simulink model "receiver_overall_v3"  (Simulink 7.5)
settings: Solver=FixedStepDiscrete  SolverMode=SingleTasking  StartTime=0.0  StopTime=(length(simin.signals.values)-1)/Fs  FixedStep=1  RelTol=1e-3
undefined symbols (not defined in the file): Fs
libraries: xbsIndex_r4 x939, symbols x8, dspsigops x2
(part 1 of 9)
settings Model: Creator=ich  LastModifiedBy=ich
settings DataIOCC: ExternalInput=simin  LimitDataPoints=off  LoadExternalInput=on

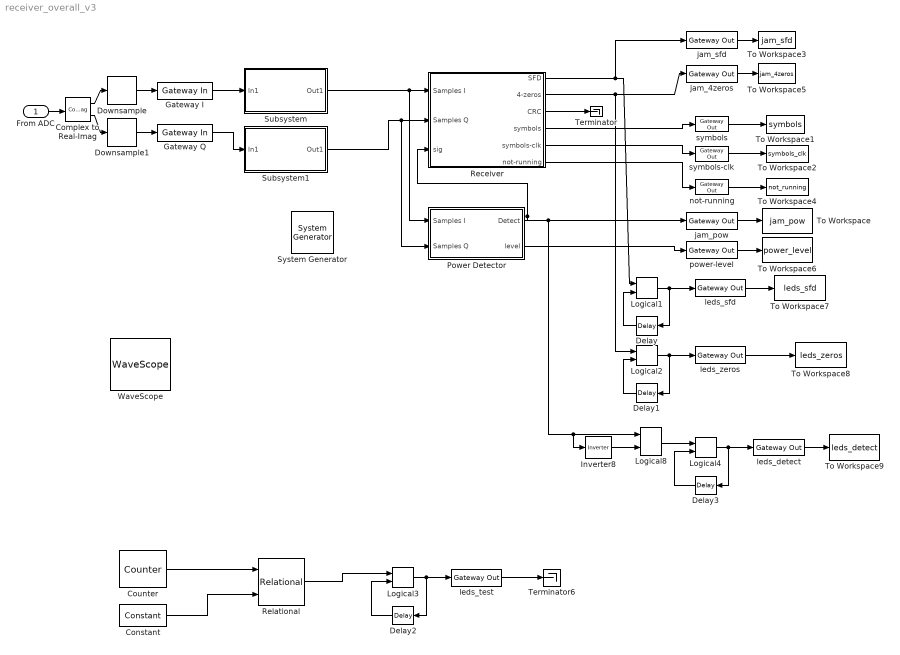
== system receiver_overall_v3 ==
  From ADC : Inport  SampleTime=1/Fs  OutDataType=fixdt(1, 16)  OutScaling=2^0  Interpolate=off
      settings: SignalType=complex
  " System Generator" : xbsIndex_r4/ System Generator  Tag=genX  SystemSampleTime=-1  xilinxfamily=spartan3  part=xc3s2000  speed=-5  package=fg456  synthesis_tool=XST  clock_wrapper=Clock Enables  directory=G:/Projekte/wireless_firewall/dschung/IEEE 802.15.4 receiver/receiver_v3  testbench=off  simulink_period=1  sysclk_period=10  dcm_input_clock_period=10  incr_netlist=off  trim_vbits=Everywhere in SubSystem  dbl_ovrd=According to Block Masks  core_generation=According to Block Masks  run_coregen=off  deprecated_control=off  eval_field=0  block_type=sysgen
      settings: block_version=12.1
  Complex to Real-Imag : ComplexToRealImag
  Constant : xbsIndex_r4/Constant  arith_type=Unsigned  const=0  n_bits=1  bin_pt=0  explicit_period=off  period=1  equ=P=C  opselect=C  inp2=PCIN>>17  opr=+  inp1=P  carry=CIN  dbl_ovrd=off  block_type=constant
      settings: block_version=12.2
  Counter : xbsIndex_r4/Counter  cnt_type=Count Limited  cnt_to=200000000  operation=Up  start_count=0  cnt_by_val=1  arith_type=Unsigned  n_bits=32  bin_pt=0  load_pin=off  rst=off  en=off  explicit_period=on  period=1  dbl_ovrd=off  use_behavioral_HDL=off  implementation=Fabric  block_type=counter
      settings: block_version=12.2
  Delay{,1..3} (4 alike) : xbsIndex_r4/Delay  en=off  latency=1  dbl_ovrd=off  reg_retiming=off  block_type=delay
      settings: block_version=12.2
  Downsample : dspsigops/Downsample  N=4  phase=0  ic=0  smode=Force single rate  fmode=Maintain input frame size
  Downsample1 : dspsigops/Downsample  N=4  phase=0  ic=0  smode=Force single rate  fmode=Maintain input frame size
  Gateway I : xbsIndex_r4/Gateway In  arith_type="Signed  (2's comp)"  n_bits=15  bin_pt=13  quantization="Round  (unbiased: +/- Inf)"  overflow=Saturate  period=1/Fs  dbl_ovrd=off  timing_constraint=None  locs_specified=off  LOCs={}  hdl_port=on  block_type=gatewayin
      settings: infoedit="Gateway in block.  Converts inputs of type Simulink integer, double and fixed point to  Xilinx fixed point type.<br><br>Hardware notes:  In hardware these blocks become top level input ports."  xl_area=[0 0 0 0 16 0 0]  block_version=12.1
  Gateway Q : xbsIndex_r4/Gateway In  arith_type="Signed  (2's comp)"  n_bits=15  bin_pt=13  quantization="Round  (unbiased: +/- Inf)"  overflow=Saturate  period=1/Fs  dbl_ovrd=off  timing_constraint=None  locs_specified=off  LOCs={}  hdl_port=on  block_type=gatewayin
      settings: infoedit="Gateway in block.  Converts inputs of type Simulink integer, double and fixed point to  Xilinx fixed point type.<br><br>Hardware notes:  In hardware these blocks become top level input ports."  xl_area=[0 0 0 0 16 0 0]  block_version=12.1
  Inverter8 : xbsIndex_r4/Inverter  en=off  latency=1  dbl_ovrd=off  block_type=inv
      settings: block_version=12.2
  Logical{1..4} (4 alike) : xbsIndex_r4/Logical  logical_function=XOR  inputs=2  en=off  latency=0  precision=Full  arith_type=Unsigned  n_bits=16  bin_pt=0  align_bp=on  dbl_ovrd=off  block_type=logical
      settings: block_version=12.2
  Logical8 : xbsIndex_r4/Logical  logical_function=AND  inputs=2  en=off  latency=0  precision=Full  arith_type=Unsigned  n_bits=16  bin_pt=0  align_bp=on  dbl_ovrd=off  block_type=logical
      settings: block_version=12.2
  Power Detector : Subsystem
  Receiver : Subsystem
  Relational : xbsIndex_r4/Relational  mode=a=b  en=off  latency=1  dbl_ovrd=off  block_type=relational
      settings: block_version=12.2
  Subsystem : Subsystem
      mask Display:
      | disp('Interpolate');
      | port_label('input',1,'in');
      | port_label('output',1,'out');
  Subsystem1 : Subsystem
      mask Display:
      | disp('Interpolate');
      | port_label('input',1,'in');
      | port_label('output',1,'out');
  Terminator : Terminator
  Terminator6 : Terminator
  To Workspace : ToWorkspace  VariableName=jam_pow  SampleTime=-1  SaveFormat=Structure
  To Workspace1 : ToWorkspace  VariableName=symbols  SampleTime=-1  SaveFormat=Structure
  To Workspace2 : ToWorkspace  VariableName=symbols_clk  SampleTime=-1  SaveFormat=Structure
  To Workspace3 : ToWorkspace  VariableName=jam_sfd  SampleTime=-1  SaveFormat=Structure
  To Workspace4 : ToWorkspace  VariableName=not_running  SampleTime=-1  SaveFormat=Structure
  To Workspace5 : ToWorkspace  VariableName=jam_4zeros  SampleTime=-1  SaveFormat=Structure
  To Workspace6 : ToWorkspace  VariableName=power_level  SampleTime=-1  SaveFormat=Structure
  To Workspace7 : ToWorkspace  VariableName=leds_sfd  SampleTime=-1  SaveFormat=Structure
  To Workspace8 : ToWorkspace  VariableName=leds_zeros  SampleTime=-1  SaveFormat=Structure
  To Workspace9 : ToWorkspace  VariableName=leds_detect  SampleTime=-1  SaveFormat=Structure
  WaveScope : xbsIndex_r4/WaveScope  block_type=wavescope
      settings: block_version=12.2
  jam_4zeros : xbsIndex_r4/Gateway Out  hdl_port=on  timing_constraint=None  locs_specified=off  LOCs={}  block_type=gatewayout
      settings: infoedit="Gateway out block.  Converts Xilinx fixed point inputs into ouputs of type Simulink integer, double, or fixed point.<br><br>Hardware notes:  In hardware these blocks become top level output ports or are discarded, depending on how they are configured."  block_version=12.2
  jam_pow : xbsIndex_r4/Gateway Out  hdl_port=on  timing_constraint=None  locs_specified=off  LOCs={}  block_type=gatewayout
      settings: infoedit="Gateway out block.  Converts Xilinx fixed point inputs into ouputs of type Simulink integer, double, or fixed point.<br><br>Hardware notes:  In hardware these blocks become top level output ports or are discarded, depending on how they are configured."  block_version=12.2
  jam_sfd : xbsIndex_r4/Gateway Out  hdl_port=on  timing_constraint=None  locs_specified=off  LOCs={}  block_type=gatewayout
      settings: infoedit="Gateway out block.  Converts Xilinx fixed point inputs into ouputs of type Simulink integer, double, or fixed point.<br><br>Hardware notes:  In hardware these blocks become top level output ports or are discarded, depending on how they are configured."  block_version=12.2
  leds_detect : xbsIndex_r4/Gateway Out  hdl_port=on  timing_constraint=None  locs_specified=off  LOCs={}  block_type=gatewayout
      settings: infoedit="Gateway out block.  Converts Xilinx fixed point inputs into ouputs of type Simulink integer, double, or fixed point.<br><br>Hardware notes:  In hardware these blocks become top level output ports or are discarded, depending on how they are configured."  block_version=12.2
  leds_sfd : xbsIndex_r4/Gateway Out  hdl_port=on  timing_constraint=None  locs_specified=off  LOCs={}  block_type=gatewayout
      settings: infoedit="Gateway out block.  Converts Xilinx fixed point inputs into ouputs of type Simulink integer, double, or fixed point.<br><br>Hardware notes:  In hardware these blocks become top level output ports or are discarded, depending on how they are configured."  block_version=12.2
  leds_test : xbsIndex_r4/Gateway Out  hdl_port=on  timing_constraint=None  locs_specified=off  LOCs={}  block_type=gatewayout
      settings: infoedit="Gateway out block.  Converts Xilinx fixed point inputs into ouputs of type Simulink integer, double, or fixed point.<br><br>Hardware notes:  In hardware these blocks become top level output ports or are discarded, depending on how they are configured."  block_version=12.2
  leds_zeros : xbsIndex_r4/Gateway Out  hdl_port=on  timing_constraint=None  locs_specified=off  LOCs={}  block_type=gatewayout
      settings: infoedit="Gateway out block.  Converts Xilinx fixed point inputs into ouputs of type Simulink integer, double, or fixed point.<br><br>Hardware notes:  In hardware these blocks become top level output ports or are discarded, depending on how they are configured."  block_version=12.2
  not-running : xbsIndex_r4/Gateway Out  hdl_port=on  timing_constraint=None  locs_specified=off  LOCs={}  block_type=gatewayout
      settings: infoedit="Gateway out block.  Converts Xilinx fixed point inputs into ouputs of type Simulink integer, double, or fixed point.<br><br>Hardware notes:  In hardware these blocks become top level output ports or are discarded, depending on how they are configured."  block_version=12.2
  power-level : xbsIndex_r4/Gateway Out  hdl_port=on  timing_constraint=None  locs_specified=off  LOCs={}  block_type=gatewayout
      settings: infoedit="Gateway out block.  Converts Xilinx fixed point inputs into ouputs of type Simulink integer, double, or fixed point.<br><br>Hardware notes:  In hardware these blocks become top level output ports or are discarded, depending on how they are configured."  block_version=12.2
  symbols : xbsIndex_r4/Gateway Out  hdl_port=on  timing_constraint=None  locs_specified=off  LOCs={}  block_type=gatewayout
      settings: infoedit="Gateway out block.  Converts Xilinx fixed point inputs into ouputs of type Simulink integer, double, or fixed point.<br><br>Hardware notes:  In hardware these blocks become top level output ports or are discarded, depending on how they are configured."  block_version=12.2
  symbols-clk : xbsIndex_r4/Gateway Out  hdl_port=on  timing_constraint=None  locs_specified=off  LOCs={}  block_type=gatewayout
      settings: infoedit="Gateway out block.  Converts Xilinx fixed point inputs into ouputs of type Simulink integer, double, or fixed point.<br><br>Hardware notes:  In hardware these blocks become top level output ports or are discarded, depending on how they are configured."  block_version=12.2
  wires:
  Gateway I/1 -> Subsystem/1(In1)
  Gateway Q/1 -> Subsystem1/1(In1)
  From ADC/1 -> Complex to Real-Imag/1
  Complex to Real-Imag/1 -> Downsample/1
  Complex to Real-Imag/2 -> Downsample1/1
  Receiver/3(CRC) -> Terminator/1
  Logical1/1 -> Delay/1, leds_sfd/1
  Delay/1 -> Logical1/2
  Logical2/1 -> Delay1/1, leds_zeros/1
  Delay1/1 -> Logical2/2
  leds_test/1 -> Terminator6/1
  Logical3/1 -> Delay2/1, leds_test/1
  Delay2/1 -> Logical3/2
  Counter/1 -> Relational/1
  Constant/1 -> Relational/2
  Relational/1 -> Logical3/1
  symbols/1 -> To Workspace1/1
  symbols-clk/1 -> To Workspace2/1
  Receiver/2(4-zeros) -> Logical2/1, jam_4zeros/1
  Receiver/1(SFD) -> Logical1/1, jam_sfd/1
  Receiver/4(symbols) -> symbols/1
  Receiver/5(symbols-clk) -> symbols-clk/1
  not-running/1 -> To Workspace4/1
  Receiver/6(not-running) -> not-running/1
  jam_4zeros/1 -> To Workspace5/1
  jam_sfd/1 -> To Workspace3/1
  Power Detector/1(Detect) -> Receiver/3(sig), jam_pow/1, Logical8/1, Inverter8/1
  jam_pow/1 -> To Workspace/1
  power-level/1 -> To Workspace6/1
  Power Detector/2(level) -> power-level/1
  Subsystem/1(Out1) -> Receiver/1(Samples I), Power Detector/1(Samples I)
  Subsystem1/1(Out1) -> Receiver/2(Samples Q), Power Detector/2(Samples Q)
  Downsample/1 -> Gateway I/1
  Downsample1/1 -> Gateway Q/1
  leds_sfd/1 -> To Workspace7/1
  leds_zeros/1 -> To Workspace8/1
  Inverter8/1 -> Logical8/2
  Logical4/1 -> Delay3/1, leds_detect/1
  Logical8/1 -> Logical4/1
  Delay3/1 -> Logical4/2
  leds_detect/1 -> To Workspace9/1

== system receiver_overall_v3/Power Detector ==
  note: 14bit signed * 14bit signed = 29bit unsigned
      | but one bit only for 10...0 * 10...0 is too expensive -> 28bit
  Samples I : Inport
  Samples Q : Inport  Port=2
  -3dB : xbsIndex_r4/Constant  arith_type=Unsigned  const=0.5  n_bits=16  bin_pt=16  explicit_period=off  period=1  equ=P=C  opselect=C  inp2=PCIN>>17  opr=+  inp1=P  carry=CIN  dbl_ovrd=off  block_type=constant
      settings: block_version=12.2
  AddSub : xbsIndex_r4/AddSub  mode=Addition  use_carryin=off  use_carryout=off  en=off  latency=0  precision=Full  arith_type=Unsigned  n_bits=16  bin_pt=14  quantization=Truncate  overflow=Wrap  dbl_ovrd=off  use_behavioral_HDL=off  hw_selection=Fabric  pipelined=off  block_type=addsub
      settings: block_version=12.2
  Convert : xbsIndex_r4/Convert  arith_type="Signed  (2's comp)"  n_bits=14  bin_pt=12  quantization=Truncate  overflow=Wrap  en=off  latency=0  dbl_ovrd=off  pipeline=off  block_type=convert
      settings: block_version=12.2
  Convert1 : xbsIndex_r4/Convert  arith_type="Signed  (2's comp)"  n_bits=14  bin_pt=12  quantization=Truncate  overflow=Wrap  en=off  latency=0  dbl_ovrd=off  pipeline=off  block_type=convert
      settings: block_version=12.2
  Moving Average : Subsystem
  Mult : xbsIndex_r4/Mult  precision=User Defined  arith_type=Unsigned  n_bits=28  bin_pt=26  quantization=Truncate  overflow=Wrap  en=off  latency=4  dbl_ovrd=off  use_behavioral_HDL=off  opt=Speed  use_embedded=off  optimum_pipeline=on  pipeline=on  use_rpm=on  placement_style=Triangular  block_type=mult
      settings: block_version=12.2
  Mult1 : xbsIndex_r4/Mult  precision=User Defined  arith_type=Unsigned  n_bits=28  bin_pt=26  quantization=Truncate  overflow=Wrap  en=off  latency=4  dbl_ovrd=off  use_behavioral_HDL=off  opt=Speed  use_embedded=off  optimum_pipeline=on  pipeline=on  use_rpm=on  placement_style=Triangular  block_type=mult
      settings: block_version=12.2
  Relational2 : xbsIndex_r4/Relational  mode=a>b  en=off  latency=1  dbl_ovrd=off  block_type=relational
      settings: block_version=12.2
  Detect : Outport
  level : Outport  Port=2
  wires:
  Samples Q/1 -> Convert1/1
  Relational2/1 -> Detect/1
  Samples I/1 -> Convert/1
  Mult/1 -> AddSub/1
  Mult1/1 -> AddSub/2
  AddSub/1 -> Moving Average/1(in)
  -3dB/1 -> Relational2/2
  Moving Average/1(short) -> Relational2/1, level/1
  Convert/1 -> Mult/1, Mult/2
  Convert1/1 -> Mult1/2, Mult1/1

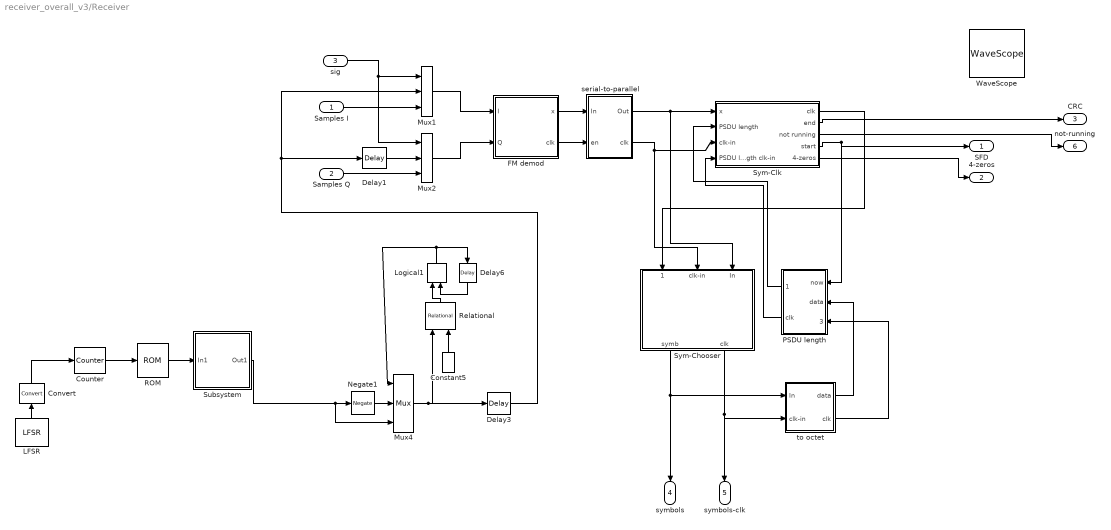
== system receiver_overall_v3/Receiver ==
  Samples I : Inport  SampleTime=1/Fs  OutDataType=fixdt(1, 16)  OutScaling=2^0  Interpolate=off
  Samples Q : Inport  Port=2  SampleTime=1/Fs  OutDataType=fixdt(1, 16)  OutScaling=2^0  Interpolate=off
  sig : Inport  Port=3  OutDataType=fixdt(1, 16)  OutScaling=2^0
  Constant5 : xbsIndex_r4/Constant  arith_type=Unsigned  const=0  n_bits=1  bin_pt=0  explicit_period=on  period=1  equ=P=C  opselect=C  inp2=PCIN>>17  opr=+  inp1=P  carry=CIN  dbl_ovrd=off  block_type=constant
      settings: block_version=12.2
  Convert : xbsIndex_r4/Convert  arith_type=Boolean  n_bits=16  bin_pt=14  quantization=Truncate  overflow=Wrap  en=off  latency=0  dbl_ovrd=off  pipeline=off  block_type=convert
      settings: block_version=12.2
  Counter : xbsIndex_r4/Counter  cnt_type=Count Limited  cnt_to=24  operation=Up  start_count=0  cnt_by_val=1  arith_type=Unsigned  n_bits=5  bin_pt=0  load_pin=off  rst=off  en=on  explicit_period=on  period=1  dbl_ovrd=off  use_behavioral_HDL=off  implementation=Fabric  block_type=counter
      settings: block_version=12.2
  Delay1 : xbsIndex_r4/Delay  en=off  latency=50  dbl_ovrd=off  reg_retiming=off  block_type=delay
      settings: block_version=12.2
  Delay3 : xbsIndex_r4/Delay  en=off  latency=30  dbl_ovrd=off  reg_retiming=off  block_type=delay
      settings: block_version=12.2
  Delay6 : xbsIndex_r4/Delay  en=off  latency=1  dbl_ovrd=off  reg_retiming=off  block_type=delay
      settings: block_version=12.2
  FM demod : Subsystem
      mask Display:
      | disp('FM\ndemod');
      | port_label('input',1,'I');
      | port_label('input',2,'Q');
      | port_label('output',1,'x');
      | port_label('output',2,'clk');
  LFSR : xbsIndex_r4/LFSR  lfsr_type=Fibonacci  gate_type=XOR  n_bits=4  polynomial='1'  rst_value='1'  rst=off  en=off  reloadable_seed=off  input_type=off  output_type=off  arith_type="Signed  (2's comp)"  bin_pt=4  dbl_ovrd=off  explicit_period=off  period=1  block_type=lfsr
      settings: block_version=12.2
  Logical1 : xbsIndex_r4/Logical  logical_function=XOR  inputs=2  en=off  latency=0  precision=Full  arith_type=Unsigned  n_bits=16  bin_pt=0  align_bp=on  dbl_ovrd=off  block_type=logical
      settings: block_version=12.2
  Mux1 : xbsIndex_r4/Mux  inputs=2  en=off  latency=0  precision=User Defined  arith_type="Signed  (2's comp)"  n_bits=15  bin_pt=13  quantization=Truncate  overflow=Wrap  dbl_ovrd=off  block_type=mux
      settings: block_version=12.2
  Mux2 : xbsIndex_r4/Mux  inputs=2  en=off  latency=0  precision=User Defined  arith_type="Signed  (2's comp)"  n_bits=15  bin_pt=13  quantization=Truncate  overflow=Wrap  dbl_ovrd=off  block_type=mux
      settings: block_version=12.2
  Mux4 : xbsIndex_r4/Mux  inputs=2  en=off  latency=0  precision=Full  arith_type=Unsigned  n_bits=16  bin_pt=14  quantization=Truncate  overflow=Wrap  dbl_ovrd=off  block_type=mux
      settings: block_version=12.2
  Negate1 : xbsIndex_r4/Negate  precision=Full  arith_type="Signed  (2's comp)"  n_bits=16  bin_pt=14  quantization=Truncate  overflow=Wrap  en=off  latency=0  dbl_ovrd=off  block_type=negate
      settings: block_version=12.2
  PSDU length : Subsystem
  ROM : xbsIndex_r4/ROM  depth=25  initVector=sin(pi*(0:4:99)/100)  distributed_mem=Distributed memory  rst=off  init_reg=0  en=off  latency=2  arith_type=Unsigned  n_bits=14  bin_pt=13  dbl_ovrd=off  optimize=Area  use_rpm=on  block_type=sprom
      settings: block_version=12.2
  Relational : xbsIndex_r4/Relational  mode=a=b  en=off  latency=1  dbl_ovrd=off  block_type=relational
      settings: block_version=12.2
  Subsystem : Subsystem
      mask Display:
      | disp('Interpolate');
      | port_label('input',1,'in');
      | port_label('output',1,'out');
  Sym-Chooser : Subsystem
  Sym-Clk : Subsystem
  WaveScope : xbsIndex_r4/WaveScope  block_type=wavescope
      settings: block_version=12.2
  serial-to-parallel : Subsystem
      mask init:
      | % save_gcb = gcb
      | % nbits=bits+1
      | % old=find_system(save_gcb,...
      | %     'lookUnderMasks', 'all',...
      | %     'RegExp', 'On',...
      | %     'Name', 'DE\d+');
      | % 
      | %     for i=1:length(old)-1
      | %         delete_line(gcb, ['DE' int2str(i) '/1'], ['DE' int2str(i+1) '/1']);
      | %     end
      | %     for i=1:length(old)
      | %         delete_line(gcb, ['DE' int2str(i) '/2'], ['Concat/' int2str(length(old)-i+1)]);
      | %     end
      | %     delete_line(gcb, '1to2/2', ['Concat/', int2str(length(old)+1)]);
      | %     delete_line(gcb, ['DE' int2str(length(old)) '/1'], ['Terminator/1']);
      | %     for i=2:length(old)
      | %         delete_block(old{i});
      | %     end
      | % 
      | % pos = get_param([save_gcb '/DE1'], 'Position');
      | % width = pos(3)-pos(1);
      | % for i=3:nbits,
      | %     add_block([save_gcb '/DE1'],[save_gcb '/DE' int2str(i-1)],'position',[pos(1)+2*(i-2)*width, pos(2), pos(3)+2*(i-2)*width, pos(4)]);
      | %     add_line(save_gcb, ['DE' int2str(i-2) '/1'], ['DE' int2str(i-1) '/1'], 'autorouting', 'on');    
      | % end
      | % 
      | % posT = get_param([save_gcb '/Terminator'], 'Position');
      | % widthT = posT(3)-posT(1);
      | % heightT = posT(4)-posT(2);
      | % set_param([save_gcb '/Terminator'], 'Position', [pos(1)+2*(nbits-1)*width pos(2) pos(1)+2*(nbits-1)*width+widthT pos(2)+heightT]);
      | % 
      | % add_line(save_gcb, ['DE' int2str(nbits-1) '/1'], ['Terminator/1'], 'autorouting', 'on');
      | % 
      | % posC = get_param([save_gcb '/Concat'], 'Position');
      | % set_param([save_gcb '/Concat'], 'Position', [pos(1)+2*(nbits)*width posC(2) pos(1)+2*(nbits+1)*width posC(2)+2*(nbits-1)*width]);
      | % set_param([save_gcb '/Concat'], 'num_inputs', int2str(nbits));
      | % 
      | % add_line(save_gcb, '1to2/2', ['Concat/' int2str(nbits)], 'autorouting', 'on');
      | % for i=1:nbits-1,
      | %    add_line(save_gcb, ['DE' int2str(i) '/2'], ['Concat/' int2str(nbits-i)], 'autorouting', 'on');
      | % end
  to octet : Subsystem
  SFD : Outport  OutDataType=fixdt(1, 16)  OutScaling=2^0
  4-zeros : Outport  Port=2  OutDataType=fixdt(1, 16)  OutScaling=2^0
  CRC : Outport  Port=3  OutDataType=fixdt(1, 16)  OutScaling=2^0
  symbols : Outport  Port=4  OutDataType=fixdt(1, 16)  OutScaling=2^0
  symbols-clk : Outport  Port=5  OutDataType=fixdt(1, 16)  OutScaling=2^0
  not-running : Outport  Port=6  OutDataType=fixdt(1, 16)  OutScaling=2^0
  wires:
  Sym-Clk/1(clk) -> Sym-Chooser/1(clk-symb-in)
  PSDU length/1(length) -> Sym-Clk/2(PSDU length)
  Sym-Clk/2(end) -> CRC/1
  Sym-Chooser/1(symb) -> to octet/1(In), symbols/1
  FM demod/1(x) -> serial-to-parallel/1(In)
  serial-to-parallel/1(Out) -> Sym-Clk/1(x), Sym-Chooser/3(In)
  Sym-Clk/4(start) -> PSDU length/1(now), SFD/1
  Sym-Clk/3(not running) -> not-running/1
  FM demod/2(clk) -> serial-to-parallel/2(en)
  serial-to-parallel/2(clk) -> Sym-Clk/3(clk-in), Sym-Chooser/2(clk-in)
  Samples I/1 -> Mux1/3
  Samples Q/1 -> Mux2/3
  sig/1 -> Mux1/1, Mux2/1
  Mux1/1 -> FM demod/1(I)
  Mux2/1 -> FM demod/2(Q)
  Sym-Chooser/2(clk) -> to octet/2(clk-in), symbols-clk/1
  to octet/1(data) -> PSDU length/2(data)
  to octet/2(clk) -> PSDU length/3(clk-in)
  PSDU length/2(clk) -> Sym-Clk/4(PSDU length clk-in)
  Sym-Clk/5(4-zeros) -> 4-zeros/1
  Delay1/1 -> Mux2/2
  Counter/1 -> ROM/1
  Subsystem/1(Out1) -> Negate1/1, Mux4/3
  Mux4/1 -> Relational/1, Delay3/1
  Constant5/1 -> Relational/2
  Relational/1 -> Logical1/1
  Logical1/1 -> Delay6/1, Mux4/1
  Delay6/1 -> Logical1/2
  Negate1/1 -> Mux4/2
  LFSR/1 -> Convert/1
  Convert/1 -> Counter/1
  Delay3/1 -> Delay1/1, Mux1/2
  ROM/1 -> Subsystem/1(In1)

== system receiver_overall_v3/Subsystem ==
  In1 : Inport
  AddSub1 : xbsIndex_r4/AddSub  mode=Addition  use_carryin=off  use_carryout=off  en=off  latency=0  precision=Full  arith_type=Unsigned  n_bits=16  bin_pt=14  quantization=Truncate  overflow=Wrap  dbl_ovrd=off  use_behavioral_HDL=off  hw_selection=Fabric  pipelined=off  block_type=addsub
      settings: block_version=12.2
  AddSub2 : xbsIndex_r4/AddSub  mode=Addition  use_carryin=off  use_carryout=off  en=off  latency=0  precision=Full  arith_type=Unsigned  n_bits=16  bin_pt=14  quantization=Truncate  overflow=Wrap  dbl_ovrd=off  use_behavioral_HDL=off  hw_selection=Fabric  pipelined=off  block_type=addsub
      settings: block_version=12.2
  AddSub3 : xbsIndex_r4/AddSub  mode=Addition  use_carryin=off  use_carryout=off  en=off  latency=1  precision=Full  arith_type=Unsigned  n_bits=16  bin_pt=14  quantization=Truncate  overflow=Wrap  dbl_ovrd=off  use_behavioral_HDL=off  hw_selection=Fabric  pipelined=off  block_type=addsub
      settings: block_version=12.2
  Convert : xbsIndex_r4/Convert  arith_type="Signed  (2's comp)"  n_bits=15  bin_pt=13  quantization=Truncate  overflow=Wrap  en=off  latency=0  dbl_ovrd=off  pipeline=off  block_type=convert
      settings: block_version=12.2
  Delay2 : xbsIndex_r4/Delay  en=off  latency=1  dbl_ovrd=off  reg_retiming=off  block_type=delay
      settings: block_version=12.2
  Delay4 : xbsIndex_r4/Delay  en=off  latency=1  dbl_ovrd=off  reg_retiming=off  block_type=delay
      settings: block_version=12.2
  Delay5 : xbsIndex_r4/Delay  en=off  latency=1  dbl_ovrd=off  reg_retiming=off  block_type=delay
      settings: block_version=12.2
  Reinterpret : xbsIndex_r4/Reinterpret  force_arith_type=off  arith_type=Unsigned  force_bin_pt=on  bin_pt=15  block_type=reinterpret
      settings: infoedit="Changes signal type without altering the binary representation.   You can changed the signal between signed and unsigned, and relocate the binary point.<br><br>Hardware notes: In hardware this block costs nothing.<br><br>Example:  Suppose the input is 6 bits wide, signed, with 2 fractional bits, and the output is forced to unsigned with 0 fractional bits.  Then an input of -2.0 (1110.00 in binary 2's complement) becomes an output of 56 (111000 in binary)."  block_version=12.2
  Out1 : Outport
  wires:
  In1/1 -> Delay2/1, AddSub1/1
  Delay2/1 -> AddSub1/2, Delay4/1
  Delay4/1 -> AddSub2/1, Delay5/1
  Delay5/1 -> AddSub2/2
  AddSub1/1 -> AddSub3/1
  AddSub2/1 -> AddSub3/2
  AddSub3/1 -> Reinterpret/1
  Reinterpret/1 -> Convert/1
  Convert/1 -> Out1/1

== system receiver_overall_v3/Subsystem1 ==
  In1 : Inport
  AddSub1 : xbsIndex_r4/AddSub  mode=Addition  use_carryin=off  use_carryout=off  en=off  latency=0  precision=Full  arith_type=Unsigned  n_bits=16  bin_pt=14  quantization=Truncate  overflow=Wrap  dbl_ovrd=off  use_behavioral_HDL=off  hw_selection=Fabric  pipelined=off  block_type=addsub
      settings: block_version=12.2
  AddSub2 : xbsIndex_r4/AddSub  mode=Addition  use_carryin=off  use_carryout=off  en=off  latency=0  precision=Full  arith_type=Unsigned  n_bits=16  bin_pt=14  quantization=Truncate  overflow=Wrap  dbl_ovrd=off  use_behavioral_HDL=off  hw_selection=Fabric  pipelined=off  block_type=addsub
      settings: block_version=12.2
  AddSub3 : xbsIndex_r4/AddSub  mode=Addition  use_carryin=off  use_carryout=off  en=off  latency=1  precision=Full  arith_type=Unsigned  n_bits=16  bin_pt=14  quantization=Truncate  overflow=Wrap  dbl_ovrd=off  use_behavioral_HDL=off  hw_selection=Fabric  pipelined=off  block_type=addsub
      settings: block_version=12.2
  Convert : xbsIndex_r4/Convert  arith_type="Signed  (2's comp)"  n_bits=15  bin_pt=13  quantization=Truncate  overflow=Wrap  en=off  latency=0  dbl_ovrd=off  pipeline=off  block_type=convert
      settings: block_version=12.2
  Delay2 : xbsIndex_r4/Delay  en=off  latency=1  dbl_ovrd=off  reg_retiming=off  block_type=delay
      settings: block_version=12.2
  Delay4 : xbsIndex_r4/Delay  en=off  latency=1  dbl_ovrd=off  reg_retiming=off  block_type=delay
      settings: block_version=12.2
  Delay5 : xbsIndex_r4/Delay  en=off  latency=1  dbl_ovrd=off  reg_retiming=off  block_type=delay
      settings: block_version=12.2
  Reinterpret : xbsIndex_r4/Reinterpret  force_arith_type=off  arith_type=Unsigned  force_bin_pt=on  bin_pt=15  block_type=reinterpret
      settings: infoedit="Changes signal type without altering the binary representation.   You can changed the signal between signed and unsigned, and relocate the binary point.<br><br>Hardware notes: In hardware this block costs nothing.<br><br>Example:  Suppose the input is 6 bits wide, signed, with 2 fractional bits, and the output is forced to unsigned with 0 fractional bits.  Then an input of -2.0 (1110.00 in binary 2's complement) becomes an output of 56 (111000 in binary)."  block_version=12.2
  Out1 : Outport
  wires:
  In1/1 -> Delay2/1, AddSub1/1
  Delay2/1 -> AddSub1/2, Delay4/1
  Delay4/1 -> AddSub2/1, Delay5/1
  Delay5/1 -> AddSub2/2
  AddSub1/1 -> AddSub3/1
  AddSub2/1 -> AddSub3/2
  AddSub3/1 -> Reinterpret/1
  Reinterpret/1 -> Convert/1
  Convert/1 -> Out1/1

== system receiver_overall_v3/Power Detector/Moving Average ==
  in : Inport
  AddSub1 : xbsIndex_r4/AddSub  mode=Addition  use_carryin=off  use_carryout=off  en=off  latency=1  precision=User Defined  arith_type="Signed  (2's comp)"  n_bits=39  bin_pt=31  quantization=Truncate  overflow=Wrap  dbl_ovrd=off  use_behavioral_HDL=off  hw_selection=Fabric  pipelined=off  block_type=addsub
      settings: block_version=12.2
  AddSub2 : xbsIndex_r4/AddSub  mode=Subtraction  use_carryin=off  use_carryout=off  en=off  latency=0  precision=Full  arith_type=Unsigned  n_bits=16  bin_pt=14  quantization=Truncate  overflow=Wrap  dbl_ovrd=off  use_behavioral_HDL=off  hw_selection=Fabric  pipelined=off  block_type=addsub
      settings: block_version=12.2
  Convert : xbsIndex_r4/Convert  arith_type="Signed  (2's comp)"  n_bits=31  bin_pt=31  quantization=Truncate  overflow=Wrap  en=off  latency=0  dbl_ovrd=off  pipeline=off  block_type=convert
      settings: block_version=12.2
  Delay1 : xbsIndex_r4/Delay  en=off  latency=32  dbl_ovrd=off  reg_retiming=off  block_type=delay
      settings: block_version=12.2
  Down Sample : xbsIndex_r4/Down Sample  sample_ratio=6  sample_phase="Last Value of Frame  (most efficient)"  en=off  latency=1  dbl_ovrd=off  block_type=dsamp
      settings: block_version=12.2
  Reinterpret : xbsIndex_r4/Reinterpret  force_arith_type=off  arith_type=Unsigned  force_bin_pt=on  bin_pt=31  block_type=reinterpret
      settings: infoedit="Changes signal type without altering the binary representation.   You can changed the signal between signed and unsigned, and relocate the binary point.<br><br>Hardware notes: In hardware this block costs nothing.<br><br>Example:  Suppose the input is 6 bits wide, signed, with 2 fractional bits, and the output is forced to unsigned with 0 fractional bits.  Then an input of -2.0 (1110.00 in binary 2's complement) becomes an output of 56 (111000 in binary)."  block_version=12.2
  Up Sample : xbsIndex_r4/Up Sample  sample_ratio=6  copy_samples=on  en=off  latency=0  dbl_ovrd=off  block_type=usamp
      settings: block_version=12.2
  short : Outport
  wires:
  in/1 -> Down Sample/1
  Delay1/1 -> AddSub2/2
  AddSub2/1 -> Convert/1
  AddSub1/1 -> Up Sample/1, AddSub1/2
  Reinterpret/1 -> AddSub1/1
  Down Sample/1 -> Delay1/1, AddSub2/1
  Up Sample/1 -> short/1
  Convert/1 -> Reinterpret/1

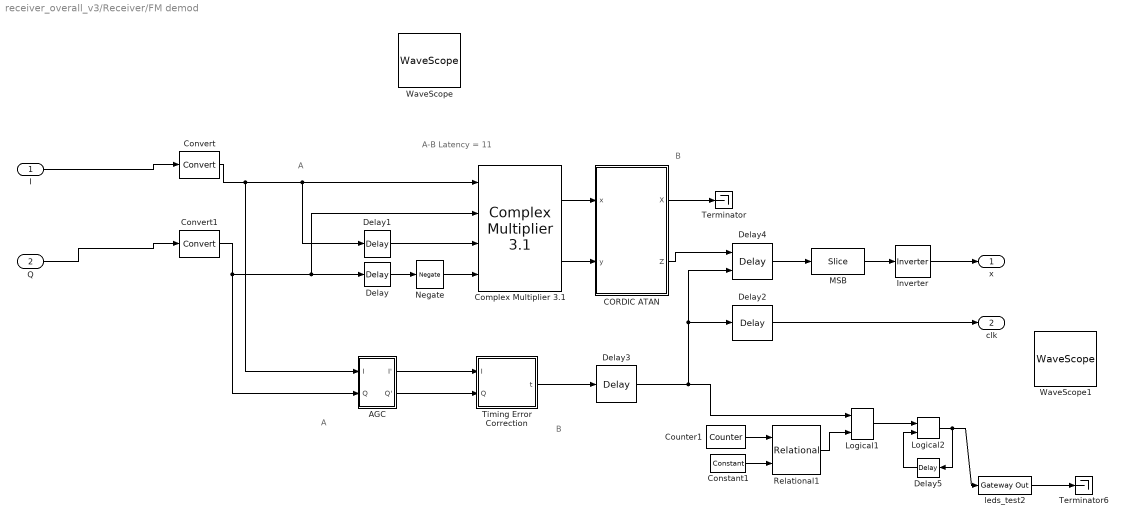
== system receiver_overall_v3/Receiver/FM demod ==
  note: A-B Latency = 11
  note: A
  note: B
  note: A
  note: B
  I : Inport
  Q : Inport  Port=2
  AGC : Subsystem
  CORDIC ATAN : Subsystem  mask(Xilinx CORDIC ATAN){stages=5, pe_nbits=33, pe_binpt=28, pipeline_x=ones(1,5), prev_stages=5, pipeline=[1  1  1  1  1]}
      mask prompts: stages "Number of Processing Elements (integer value starting from 1)"; pe_nbits "X, Y Data Width"; pe_binpt "X, Y Binary Point Position"; pipeline_x "Latency for each Processing Element [1 0 0 1]"; prev_stages "Previous Number of Stages"; pipeline "Previous Pipeline Values"
      mask help: A parallel implementation, circular vectoring mode CORDIC processor for performing rectangular-to-polar conversion. The number of iteration stages (and resultant output accuracy) and the processor arithmetic precision are controlled by the mask customization.
      mask init:
      | [bg,fg] = xlcmap('XBlock',0);
      | iPos = get_param(gcb,'Position');
      | iWidth=iPos(3)-iPos(1); iHeight=iPos(4)-iPos(2);
      | iCx=iWidth/2;
      | iCy=iHeight/2;
      | [logoX, logoY] = xlogo(iPos);
      | sav_gcb=gcb;
      | stages = round(sum(abs(stages)));
      | if (stages == 0)
      | 	stages = prev_stages;
      | end
      | x = zeros(1,stages);
      | pipe_size = max(size(pipeline_x));
      | if pipe_size >= stages
      | 	x(1,1:stages) = pipeline_x(1,1:stages);
      | else
      | 	x(1,1:pipe_size) = pipeline_x(1,1:pipe_size);
      | end
      | 
      | if (stages ~=prev_stages)
      | 	pipeline=x;
      | 	cordic_pe = find_system(gcb, 'lookUnderMasks', 'all', 'FollowLinks','on','masktype', 'CORDIC parallel PE');
      |     
      |   a=find_system(cordic_pe{1}, 'lookUnderMasks', 'all', 'FollowLinks','on','masktype', 'CORDIC iteration PE');
      |   for i= 2:length(a)
      |     for j=1:3
      | 	  delete_line(cordic_pe{1}, ['CORDIC PE' int2str(i-1) '/' int2str(j)], ['CORDIC PE' int2str(i) '/' int2str(j)]);
      |     end
      |   end
      |     if length(a)>0,
      |       delete_line(cordic_pe{1}, 'x/1', 'CORDIC PE1/1');
      |       delete_line(cordic_pe{1}, 'y/1', 'CORDIC PE1/2');
      |       delete_line(cordic_pe{1}, 'z/1', 'CORDIC PE1/3');
      |       delete_line(cordic_pe{1}, ['CORDIC PE' int2str(length(a)) '/1'],'X/1');
      |       delete_line(cordic_pe{1}, ['CORDIC PE' int2str(length(a)) '/2'],'Terminator/1');
      |       delete_line(cordic_pe{1}, ['CORDIC PE' int2str(length(a)) '/3'],'Z/1');
      |     elseif length(a)==0
      |       temp_port=get_param([cordic_pe{1} '/x'],'porthandles');
      |       temp_line=get_param(temp_port.Outport,'line');
      |       if temp_line>=0  delete_line(temp_line); end
      |       temp_port=get_param([cordic_pe{1} '/y'],'porthandles');
      |       temp_line=get_param(temp_port.Outport,'line');
      |       if temp_line>=0  delete_line(temp_line); end
      |       temp_port=get_param([cordic_pe{1} '/z'],'porthandles');
      |       temp_line=get_param(temp_port.Outport,'line');
      |       if temp_line>=0  delete_line(temp_line); end
      |     end
      | 
      |     for i=2:length(a)
      |       delete_block(a{i});
      |     end
      |     for i=2:stages,
      |         add_block([cordic_pe{1} '/CORDIC PE1'], [cordic_pe{1} '/CORDIC PE' int2str(i)], 'ii', int2str(i-1),'pe_nbits', 'pe_nbits','pe_binpt', 'pe_binpt','pipeline',['pipeline(1,' int2str(i) ')'],'position',[150+(i-1)*125, 70, 205+(i-1)*125, 130]);
      |     end
      | 
      |     for i= 2:stages,
      |       for j=1:3
      | 		add_line(cordic_pe{1}, ['CORDIC PE' int2str(i-1) '/' int2str(j)], ['CORDIC PE' int2str(i) '/' int2str(j)], 'autorouting', 'on');
      |       end
      |     end
      | 
      |     if stages==0
      |       add_line(cordic_pe{1}, 'x/1', 'X/1', 'autorouting', 'on');
      |       add_line(cordic_pe{1}, 'y/1', 'Terminator/1', 'autorouting', 'on');
      |       add_line(cordic_pe{1}, 'z/1', 'Z/1', 'autorouting', 'on');
      |     elseif stages>0
      |       add_line(cordic_pe{1}, 'x/1', 'CORDIC PE1/1', 'autorouting', 'on');
      |       add_line(cordic_pe{1}, 'y/1', 'CORDIC PE1/2', 'autorouting', 'on');
      |       add_line(cordic_pe{1}, 'z/1', 'CORDIC PE1/3', 'autorouting', 'on');
      | 
      |       set_param([cordic_pe{1} '/' 'X'], 'Position', [150+stages*125, 72, 180+stages*125, 86]);
      |       set_param([cordic_pe{1} '/' 'Terminator'], 'Position', [210+stages*125, 92, 225+stages*125, 108]);
      |       set_param([cordic_pe{1} '/' 'Z'], 'Position', [240+stages*125, 113, 270+stages*125, 127]);
      | 
      |       add_line(cordic_pe{1}, ['CORDIC PE' int2str(stages) '/1'], 'X/1', 'autorouting', 'on');
      |       add_line(cordic_pe{1}, ['CORDIC PE' int2str(stages) '/2'], 'Terminator/1', 'autorouting', 'on');
      |       add_line(cordic_pe{1}, ['CORDIC PE' int2str(stages) '/3'],'Z/1', 'autorouting', 'on');
      | 
      |       % force a "compile" of the constituent constant blocks to
      |       % workaround a data propagation problem
      |       find_system(cordic_pe{1}, 'lookUnderMasks', 'all', 'FollowLinks', 'on', 'MaskType','Xilinx Constant Block');
      |   end
      | 	set_param(sav_gcb, 'prev_stages', int2str(stages));
      | 	set_param(sav_gcb, 'pipeline', [ '[' int2str(x) ']']);
      | else
      | 	if (sum(pipeline~=x))
      | 		set_param(gcb, 'pipeline', [ '[' int2str(x) ']']);
      | 	end
      | end
      | str = sprintf('-%d',sum(x) + 3);
      settings: CopyFcn=set_param(gcb, 'MaskSelfModifiable', 'on', 'LinkStatus', 'none');
      mask Help: eval('');xlDoc('-book','sysgen','-topic','CORDIC_ATAN');
      mask Display:
      | patch([0 iWidth iWidth 0],[0 0 iHeight iHeight] , bg);
      | patch(logoX,logoY , fg);
      | text(iCx-6,iCy,'z');
      | text(iCx,iCy+4,str);
      | port_label('input',1,'I');
      | port_label('input',2,'Q');
      | port_label('output',1,'mag');
      | port_label('output',2,'atan');
      | plot([0 0 iWidth iWidth 0], [0 iHeight iHeight 0 0]);
  "Complex Multiplier 3.1 " : xbsIndex_r4/Complex Multiplier 3.1   multtype=Use_Mults  optimizegoal=Performance  outputwidthhigh=32  outputwidthlow=0  latency=-1  roundmode=Truncate  clockenable=off  syncclear=off  ip_name=Complex Multiplier  ip_version=3.1  dsptool_ready=true  ipcore_usecache=true  ipcore_useipmodelcache=true  ipcore_verbose=false  ipcore_latency_parameter='latency'  wrapper_available=true  port_translation_map={ 'ce' => 'en', 'sclr' => 'rst' }  structural_sim=false  block_type=cmpy_v3_1
      settings: xl_use_area=on  xl_area=[600 1053 0 1053 0 0 0]  block_version=12.1
  Constant1 : xbsIndex_r4/Constant  arith_type=Unsigned  const=50  n_bits=6  bin_pt=0  explicit_period=off  period=1  equ=P=C  opselect=C  inp2=PCIN>>17  opr=+  inp1=P  carry=CIN  dbl_ovrd=off  block_type=constant
      settings: block_version=12.2
  Convert : xbsIndex_r4/Convert  arith_type="Signed  (2's comp)"  n_bits=16  bin_pt=14  quantization=Truncate  overflow=Wrap  en=off  latency=0  dbl_ovrd=off  pipeline=off  block_type=convert
      settings: block_version=12.2
  Convert1 : xbsIndex_r4/Convert  arith_type="Signed  (2's comp)"  n_bits=16  bin_pt=14  quantization=Truncate  overflow=Wrap  en=off  latency=0  dbl_ovrd=off  pipeline=off  block_type=convert
      settings: block_version=12.2
  Counter1 : xbsIndex_r4/Counter  cnt_type=Count Limited  cnt_to=100000000  operation=Up  start_count=0  cnt_by_val=1  arith_type=Unsigned  n_bits=32  bin_pt=0  load_pin=off  rst=off  en=off  explicit_period=on  period=1  dbl_ovrd=off  use_behavioral_HDL=off  implementation=Fabric  block_type=counter
      settings: block_version=12.2
  Delay{,1..2,5} (4 alike) : xbsIndex_r4/Delay  en=off  latency=1  dbl_ovrd=off  reg_retiming=off  block_type=delay
      Delay settings: xl_area=[8 16 0 0 0 0 0]  block_version=12.1
      Delay1 settings: xl_area=[8 16 0 0 0 0 0]  block_version=12.1
      Delay2 settings: block_version=12.2
      Delay5 settings: block_version=12.2
  Delay3 : xbsIndex_r4/Delay  en=off  latency=25  dbl_ovrd=off  reg_retiming=off  block_type=delay
      settings: block_version=12.2
  Delay4 : xbsIndex_r4/Delay  en=on  latency=1  dbl_ovrd=off  reg_retiming=off  block_type=delay
      settings: block_version=12.2
  Inverter : xbsIndex_r4/Inverter  en=off  latency=0  dbl_ovrd=off  block_type=inv
      settings: xl_area=[0 0 0 0 0 0 0]  block_version=12.1
  Logical1 : xbsIndex_r4/Logical  logical_function=AND  inputs=2  en=off  latency=0  precision=Full  arith_type=Unsigned  n_bits=16  bin_pt=0  align_bp=on  dbl_ovrd=off  block_type=logical
      settings: block_version=12.2
  Logical2 : xbsIndex_r4/Logical  logical_function=XOR  inputs=2  en=off  latency=0  precision=Full  arith_type=Unsigned  n_bits=16  bin_pt=0  align_bp=on  dbl_ovrd=off  block_type=logical
      settings: block_version=12.2
  MSB : xbsIndex_r4/Slice  nbits=1  boolean_output=off  mode=Upper Bit Location + Width  bit1=0  base1=MSB of Input  bit0=0  base0=LSB of Input  dbl_ovrd=off  block_type=slice
      settings: block_version=12.1
  Negate : xbsIndex_r4/Negate  precision=User Defined  arith_type="Signed  (2's comp)"  n_bits=16  bin_pt=14  quantization=Truncate  overflow=Wrap  en=off  latency=0  dbl_ovrd=off  block_type=negate
      settings: xl_area=[8 0 0 16 0 0 0]  block_version=12.1
  Relational1 : xbsIndex_r4/Relational  mode=a<b  en=off  latency=1  dbl_ovrd=off  block_type=relational
      settings: block_version=12.2
  Terminator : Terminator
  Terminator6 : Terminator
  Timing Error Correction : Subsystem
  WaveScope : xbsIndex_r4/WaveScope  block_type=wavescope
      settings: block_version=12.2
  WaveScope1 : xbsIndex_r4/WaveScope  block_type=wavescope
      settings: block_version=12.2
  leds_test2 : xbsIndex_r4/Gateway Out  hdl_port=on  timing_constraint=None  locs_specified=off  LOCs={}  block_type=gatewayout
      settings: infoedit="Gateway out block.  Converts Xilinx fixed point inputs into ouputs of type Simulink integer, double, or fixed point.<br><br>Hardware notes:  In hardware these blocks become top level output ports or are discarded, depending on how they are configured."  block_version=12.2
  x : Outport
  clk : Outport  Port=2
  wires:
  Delay/1 -> Negate/1
  Delay1/1 -> "Complex Multiplier 3.1 "/3
  Negate/1 -> "Complex Multiplier 3.1 "/4
  "Complex Multiplier 3.1 "/1 -> CORDIC ATAN/1(x)
  "Complex Multiplier 3.1 "/2 -> CORDIC ATAN/2(y)
  CORDIC ATAN/1(X) -> Terminator/1
  MSB/1 -> Inverter/1
  Inverter/1 -> x/1
  I/1 -> Convert/1
  Convert1/1 -> AGC/2(Q), Delay/1, "Complex Multiplier 3.1 "/2
  Delay4/1 -> MSB/1
  CORDIC ATAN/2(Z) -> Delay4/1
  Timing Error Correction/1(t) -> Delay3/1
  Q/1 -> Convert1/1
  Convert/1 -> AGC/1(I), Delay1/1, "Complex Multiplier 3.1 "/1
  Delay2/1 -> clk/1
  AGC/1(I') -> Timing Error Correction/1(I)
  AGC/2(Q') -> Timing Error Correction/2(Q)
  Delay3/1 -> Delay2/1, Delay4/2, Logical1/1
  Counter1/1 -> Relational1/1
  Constant1/1 -> Relational1/2
  Relational1/1 -> Logical1/2
  Logical2/1 -> Delay5/1, leds_test2/1
  Delay5/1 -> Logical2/2
  Logical1/1 -> Logical2/1
  leds_test2/1 -> Terminator6/1

== system receiver_overall_v3/Receiver/PSDU length ==
  now : Inport
  data : Inport  Port=2
  clk-in : Inport  Port=3
  Constant : xbsIndex_r4/Constant  arith_type=Unsigned  const=0  n_bits=5  bin_pt=0  explicit_period=off  period=1  equ=P=C  opselect=C  inp2=PCIN>>17  opr=+  inp1=P  carry=CIN  dbl_ovrd=off  block_type=constant
      settings: block_version=12.2
  Delay1 : xbsIndex_r4/Delay  en=off  latency=1  dbl_ovrd=off  reg_retiming=off  block_type=delay
      settings: block_version=12.2
  Delay2 : xbsIndex_r4/Delay  en=on  latency=3  dbl_ovrd=off  reg_retiming=off  block_type=delay
      settings: block_version=12.2
  Delay3 : xbsIndex_r4/Delay  en=off  latency=1  dbl_ovrd=off  reg_retiming=off  block_type=delay
      settings: block_version=12.2
  Inverter1 : xbsIndex_r4/Inverter  en=off  latency=1  dbl_ovrd=off  block_type=inv
      settings: block_version=12.2
  Inverter2 : xbsIndex_r4/Inverter  en=off  latency=1  dbl_ovrd=off  block_type=inv
      settings: block_version=12.2
  Logical2 : xbsIndex_r4/Logical  logical_function=OR  inputs=2  en=off  latency=0  precision=Full  arith_type=Unsigned  n_bits=16  bin_pt=0  align_bp=on  dbl_ovrd=off  block_type=logical
      settings: block_version=12.2
  Logical4 : xbsIndex_r4/Logical  logical_function=AND  inputs=2  en=off  latency=0  precision=Full  arith_type=Unsigned  n_bits=16  bin_pt=0  align_bp=on  dbl_ovrd=off  block_type=logical
      settings: block_version=12.2
  Logical5 : xbsIndex_r4/Logical  logical_function=AND  inputs=2  en=off  latency=0  precision=Full  arith_type=Unsigned  n_bits=16  bin_pt=0  align_bp=on  dbl_ovrd=off  block_type=logical
      settings: block_version=12.2
  Logical6 : xbsIndex_r4/Logical  logical_function=AND  inputs=2  en=off  latency=0  precision=Full  arith_type=Unsigned  n_bits=16  bin_pt=0  align_bp=on  dbl_ovrd=off  block_type=logical
      settings: block_version=12.2
  PSDU length : xbsIndex_r4/Mux  inputs=2  en=off  latency=0  precision=User Defined  arith_type=Unsigned  n_bits=8  bin_pt=0  quantization=Truncate  overflow=Wrap  dbl_ovrd=off  block_type=mux
      settings: block_version=12.2
  length : Outport
  clk : Outport  Port=2
  wires:
  Constant/1 -> PSDU length/2
  PSDU length/1 -> length/1
  data/1 -> Delay3/1
  Delay1/1 -> Logical2/2
  Logical2/1 -> Logical5/1
  Inverter1/1 -> Logical5/2
  Logical5/1 -> Delay1/1, Logical4/1
  Logical4/1 -> Inverter1/1, Delay2/1
  Delay2/1 -> Logical6/1, Inverter2/1
  Inverter2/1 -> Logical6/2
  clk-in/1 -> Logical4/2, Delay2/2
  now/1 -> Logical2/1
  Delay3/1 -> PSDU length/3
  Logical6/1 -> PSDU length/1, clk/1

== system receiver_overall_v3/Receiver/Subsystem ==
  In1 : Inport
  AddSub1 : xbsIndex_r4/AddSub  mode=Addition  use_carryin=off  use_carryout=off  en=off  latency=0  precision=Full  arith_type=Unsigned  n_bits=16  bin_pt=14  quantization=Truncate  overflow=Wrap  dbl_ovrd=off  use_behavioral_HDL=off  hw_selection=Fabric  pipelined=off  block_type=addsub
      settings: block_version=12.2
  AddSub2 : xbsIndex_r4/AddSub  mode=Addition  use_carryin=off  use_carryout=off  en=off  latency=0  precision=Full  arith_type=Unsigned  n_bits=16  bin_pt=14  quantization=Truncate  overflow=Wrap  dbl_ovrd=off  use_behavioral_HDL=off  hw_selection=Fabric  pipelined=off  block_type=addsub
      settings: block_version=12.2
  AddSub3 : xbsIndex_r4/AddSub  mode=Addition  use_carryin=off  use_carryout=off  en=off  latency=1  precision=Full  arith_type=Unsigned  n_bits=16  bin_pt=14  quantization=Truncate  overflow=Wrap  dbl_ovrd=off  use_behavioral_HDL=off  hw_selection=Fabric  pipelined=off  block_type=addsub
      settings: block_version=12.2
  Delay2 : xbsIndex_r4/Delay  en=off  latency=1  dbl_ovrd=off  reg_retiming=off  block_type=delay
      settings: block_version=12.2
  Delay4 : xbsIndex_r4/Delay  en=off  latency=1  dbl_ovrd=off  reg_retiming=off  block_type=delay
      settings: block_version=12.2
  Delay5 : xbsIndex_r4/Delay  en=off  latency=1  dbl_ovrd=off  reg_retiming=off  block_type=delay
      settings: block_version=12.2
  Reinterpret : xbsIndex_r4/Reinterpret  force_arith_type=off  arith_type=Unsigned  force_bin_pt=on  bin_pt=15  block_type=reinterpret
      settings: infoedit="Changes signal type without altering the binary representation.   You can changed the signal between signed and unsigned, and relocate the binary point.<br><br>Hardware notes: In hardware this block costs nothing.<br><br>Example:  Suppose the input is 6 bits wide, signed, with 2 fractional bits, and the output is forced to unsigned with 0 fractional bits.  Then an input of -2.0 (1110.00 in binary 2's complement) becomes an output of 56 (111000 in binary)."  block_version=12.2
  Out1 : Outport
  wires:
  In1/1 -> Delay2/1, AddSub1/1
  Delay2/1 -> AddSub1/2, Delay4/1
  Delay4/1 -> AddSub2/1, Delay5/1
  Delay5/1 -> AddSub2/2
  AddSub1/1 -> AddSub3/1
  AddSub2/1 -> AddSub3/2
  AddSub3/1 -> Reinterpret/1
  Reinterpret/1 -> Out1/1
